simulink model "case_68_cut_in_sn_8_dv_15_v0_20"  (R2025b)
settings: Solver=VariableStepAuto  StartTime=0.0  StopTime=10.0  RelTol=1e-3
settings Model: Creator=jdcjd  LastModifiedBy=admin

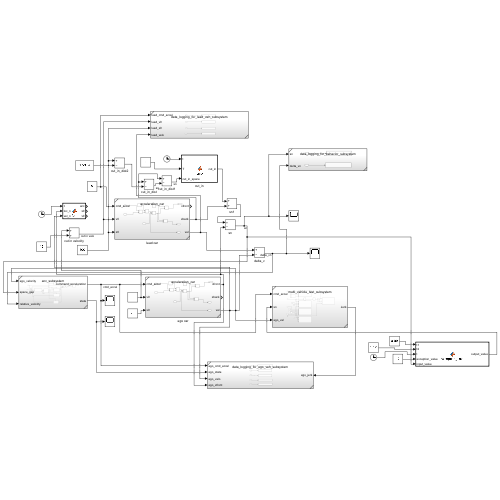
[thumbnail: Simulink's stored preview of the top-level diagram]
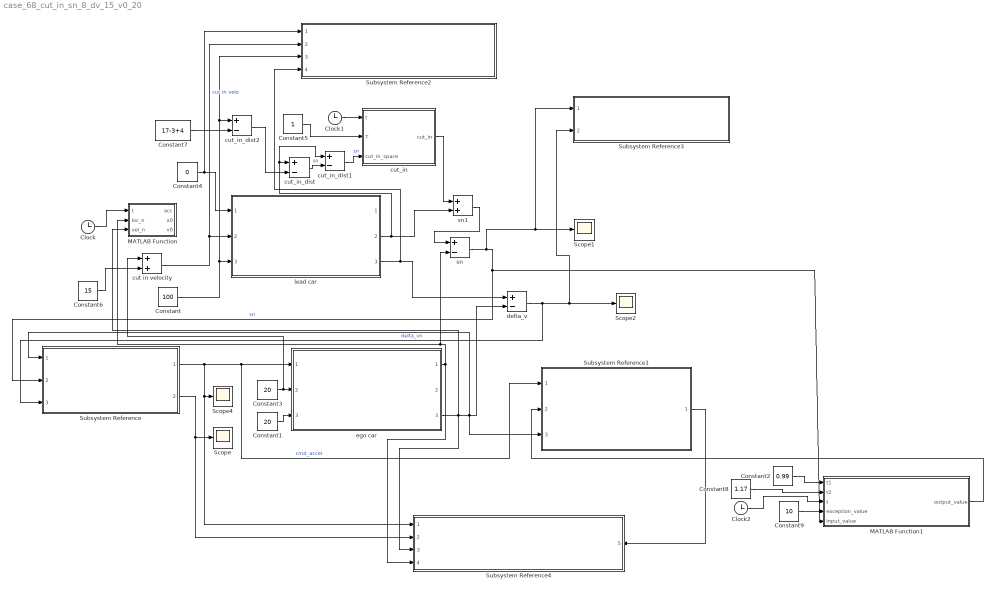
== system case_68_cut_in_sn_8_dv_15_v0_20 ==
  Clock : Clock
  Clock1 : Clock
  Clock2 : Clock
  Constant : Constant  Value=100
  Constant1 : Constant  Value=20
  Constant2 : Constant  Value=0.99
  Constant3 : Constant  Value=20
  Constant4 : Constant  Value=0
  Constant5 : Constant
  Constant6 : Constant  Value=15
  Constant7 : Constant  Value=17-3+4
  Constant8 : Constant  Value=1.17
  Constant9 : Constant  Value=10
  MATLAB Function : MATLAB Function  TreatAsAtomicUnit=on
  MATLAB Function1 : MATLAB Function  TreatAsAtomicUnit=on
  Scope{,1..2,4} (4 alike) : Scope
      Scope settings: ActiveDisplayYMinimum=-1.283115133036413  ActiveDisplayYMaximum=1.1975268354687039
      Scope1 settings: ActiveDisplayYMinimum=8.3088925580817374  ActiveDisplayYMaximum=13.206665133279719
      Scope2 settings: ActiveDisplayYMinimum=0.70692580437122388  ActiveDisplayYMaximum=33.266141389474569  DataLoggingVariableName=ScopeData2
      Scope4 settings: ActiveDisplayYMinimum=-3.920176511063207  ActiveDisplayYMaximum=2.9170461451867933  DataLoggingVariableName=ScopeData4
  Subsystem Reference : Subsystem  ReferencedSubsystem=acc_subsystem
  Subsystem Reference1 : Subsystem  ReferencedSubsystem=multi_vehicle_test_subsystem
  Subsystem Reference2 : Subsystem  ReferencedSubsystem=data_logging_for_lead_veh_subsystem
  Subsystem Reference3 : Subsystem  ReferencedSubsystem=data_logging_for_behavior_subsystem
  Subsystem Reference4 : Subsystem  ReferencedSubsystem=data_logging_for_ego_veh_subsystem
      settings: PortSchema="{\"entries\":[{\"content\":{\"sides\":[{\"content\":{\"connectorIds\":[\"In1\",\"In2\",\"In3\",\"In4\"]},\"type\":\"ConnectorPlacement.EquallySpacedRectSide\",\"uuid\":\"1bb3a8cf-f981-4f8a-aff9-03896ccf7d7c\"},{\"content\":{\"connectorIds\":[\"In5\"],\"side\":\"RIGHT\"},\"type\":\"ConnectorPlacement.EquallySpacedRectSide\",\"uuid\":\"3f6ac5cb-96be-44a3-8993-3635a91bd658\"},{\"content\":{\"side\":\"TOP\"},\"type\":\"ConnectorPlacement.EquallySpacedRectSide\",\"uuid\":\"c641fc7f-a424-4033-b273-2526f6b205c0\"}]},\"type\":\"ConnectorPlacement.EquallySpacedConnector\",\"uuid\":\"2a4be48e-084e-4aa6-b74f-8fe234fedc1a\"}],\"packageUris\":[\"http://schema.mathworks.com/mf0/Connector/R2020b\"],\"version\":\"1.0\"}"
  cut in velocity : Sum
  cut_in : MATLAB Function  TreatAsAtomicUnit=on
  cut_in_dist : Sum  Inputs=+-
  cut_in_dist1 : Sum  Inputs=+-
  cut_in_dist2 : Sum  Inputs=+-
  delta_v : Sum  Inputs=+-
  ego car : Subsystem  ReferencedSubsystem=acceleration_car
  lead car : Subsystem  ReferencedSubsystem=acceleration_car
  sn : Sum  Inputs=+-
  sn1 : Sum
  wires:
  Constant3/1 -> cut in velocity/1, ego car/2
  Constant1/1 -> ego car/3
  Clock/1 -> MATLAB Function/1(t)
  cut_in/1(cut_in) -> sn1/1
  Clock1/1 -> cut_in/1(t)
  sn1/1 -> sn/1
  Constant5/1 -> cut_in/2(T)
  delta_v/1 -> Subsystem Reference3/2, Scope2/1, Subsystem Reference/3  "delta_vn"
  Constant4/1 -> Subsystem Reference2/1, lead car/1
  lead car/3 -> Subsystem Reference2/4, delta_v/1
  sn/1 -> Scope1/1, Subsystem Reference3/1, MATLAB Function1/5(input_value), Subsystem Reference/2  "sn"
  Constant/1 -> cut_in_dist2/1, Subsystem Reference2/3, lead car/3
  ego car/3 -> Subsystem Reference4/3, MATLAB Function/3(vel_n), Subsystem Reference1/3, Subsystem Reference/1, delta_v/2
  Subsystem Reference/2 -> Subsystem Reference4/2, Scope/1
  Subsystem Reference/1 -> Scope4/1, Subsystem Reference4/1, Subsystem Reference1/1, ego car/1  "cmd_accel"
  ego car/1 -> MATLAB Function/2(loc_n), sn/2, Subsystem Reference4/4
  Subsystem Reference1/1 -> Subsystem Reference4/5
  cut_in_dist2/1 -> cut_in_dist/2
  cut_in_dist/1 -> cut_in_dist1/2  "sn"
  cut_in_dist1/1 -> cut_in/3(cut_in_space)  "sn"
  lead car/2 -> cut_in_dist1/1, cut_in_dist/1, sn1/2
  Constant7/1 -> cut_in_dist2/2
  Constant6/1 -> cut in velocity/2
  cut in velocity/1 -> Subsystem Reference2/2, lead car/2  "cut in velo"
  Constant2/1 -> MATLAB Function1/1(t1)
  Constant8/1 -> MATLAB Function1/2(t2)
  Constant9/1 -> MATLAB Function1/4(exception_value)
  Clock2/1 -> MATLAB Function1/3(t)
  MATLAB Function1/1(output_value) -> Subsystem Reference1/2

== matlab function case_68_cut_in_sn_8_dv_15_v0_20/MATLAB Function ==
  data: t input; acc output; loc_n input; vel_n input; x0 output; v0 output
function [acc, x0, v0] = fcn(t, loc_n, vel_n)

if t < 5
    acc = 0;
    x0 = 0;
    v0 = 0;
else 
    acc = 1;
    x0 = loc_n + 5;
    v0 = vel_n;

end
end

== matlab function case_68_cut_in_sn_8_dv_15_v0_20/cut_in ==
  data: t input; cut_in output; T input; cut_in_space input
function cut_in = jump(t, T, cut_in_space)
    if t < T
        cut_in = 0;
    else 
        cut_in = - cut_in_space ;
    end 
end

== matlab function case_68_cut_in_sn_8_dv_15_v0_20/MATLAB Function1 ==
  data: t1 input; t2 input; t input; exception_value input; input_value input; output_value output
function output_value = exception_time(t1, t2, t, exception_value, input_value)
if (t >= t1 ) && (t <= t2)
    output_value = exception_value;
else
    output_value = input_value;
end
